simulink model "DCAC"  (R2020b)
settings: Solver=FixedStepDiscrete  StartTime=0.0  StopTime=0.05  FixedStep=1e-8  RelTol=1e-3
PreLoadFcn:
  | addpath("Sim\");
  | run(Sim_PreLoad_DCAC.mlx);
values from neighbouring files (symbols this model uses):
  C = 1/(wl*wl*L)    [BodeCalculation.m]
  L = sqrt(((w1*(Uo_*Uo_)/(wl*wl)) + (w1*w1*w1*(Uo_*Uo_)/(wl*wl*wl*wl))) / (w1*(Io_*Io_)))    [BodeCalculation.m]    (also in draw.m = sqrt(((w1 .* (Uo_ .^ 2) / (wl * wl)) + (w1 * w1 * w1 .* (Uo_)
undefined symbols (not defined in the file or in its folder): R_Load, Ts, V_DC
libraries: powerlib x22, powerlib_meascontrol x2, simulink x1
settings Model: Creator=VanillaC  LastModifiedBy=VanillaC
settings DataIOCC: ReturnWorkspaceOutputs=off
settings OptimizationCC: DefaultParameterBehavior=Inlined  EnhancedBackFolding=on  PassReuseOutputArgsAs=Individual arguments  ZeroExternalMemoryAtStartup=off  ZeroInternalMemoryAtStartup=off  OptimizeBlockOrder=speed  DifferentSizesBufferReuse=on  OptimizationCustomize=off  EfficientTunableParamExpr=on
settings DebuggingCC: ParameterTunabilityLossMsg=error  UnconnectedInputMsg=none  UnconnectedOutputMsg=none  UnconnectedLineMsg=none
settings ModelReferenceCC: EnableRefExpFcnMdlSchedulingChecks=off
settings SFSimCC: MATLABDynamicMemAlloc=off
settings RTWCC: Description=Embedded Coder  SystemTargetFile=ert.tlc  GenCodeOnly=on  TemplateMakefile=ert_default_tmf
settings CodeAppCC: ForceParamTrailComments=on  IgnoreCustomStorageClasses=off  OperatorAnnotations=on  SimulinkDataObjDesc=on  SFDataObjDesc=on  InsertBlockDesc=on  MATLABSourceComments=on
settings ERTTargetCC: TargetLangStandard=C99 (ISO)  GenerateSampleERTMain=on  SupportContinuousTime=on  InlinedParameterPlacement=NonHierarchical  ERTCustomFileTemplate=example_file_process.tlc

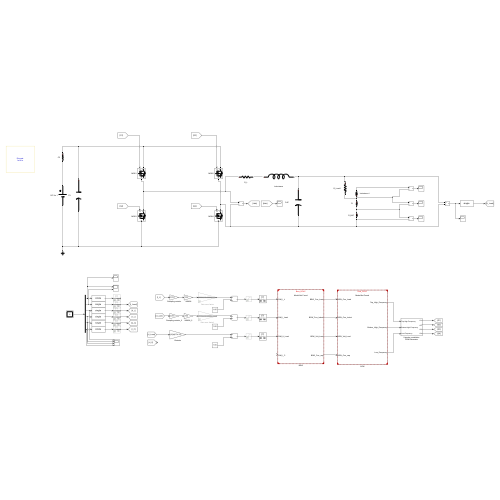
[thumbnail: Simulink's stored preview of the top-level diagram]
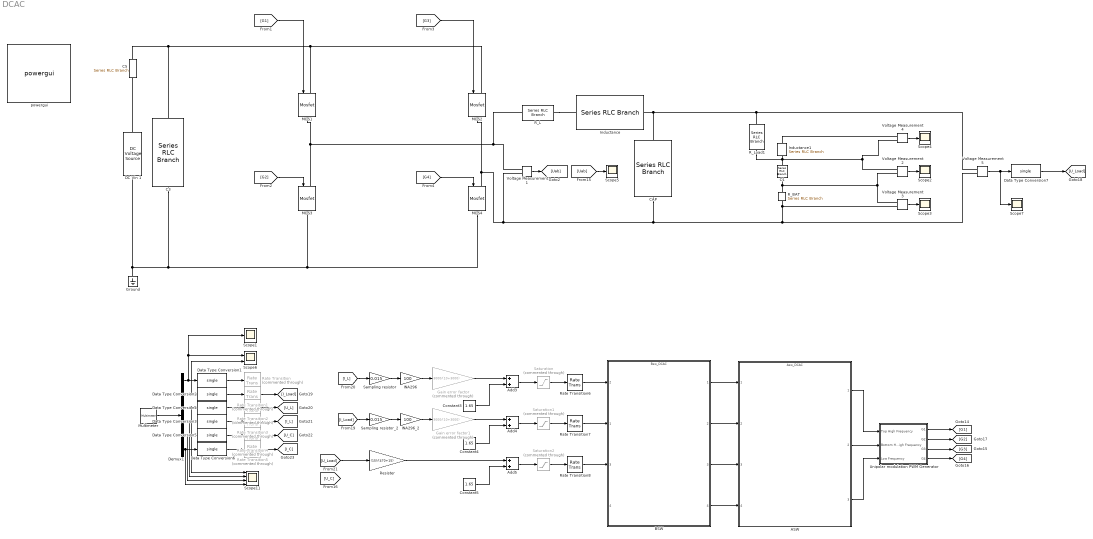
== system DCAC ==
  ASW : ModelReference  ModelNameDialog=Asw_DCAC.slx  SimulationMode=Normal  ModelReferenceVersion=1.140
  Add3 : Sum
  Add4 : Sum
  Add5 : Sum
  BSW : ModelReference  ModelNameDialog=Bsw_DCAC.slx  SimulationMode=Normal  ModelReferenceVersion=1.11
      settings: PortSchema="{\"entries\":[{\"content\":{\"sides\":[{\"content\":{\"connectorIds\":[\"In2\",\"In1\",\"In3\",\"In4\"]},\"type\":\"ConnectorPlacement.EquallySpacedRectSide\",\"uuid\":\"b2b7a57c-7cf1-4c06-9e54-7dc01d62324f\"},{\"content\":{\"connectorIds\":[\"Out1\",\"Out2\",\"Out3\",\"Out4\"],\"side\":\"RIGHT\"},\"type\":\"ConnectorPlacement.EquallySpacedRectSide\",\"uuid\":\"58967db2-deee-4275-8865-8f1f6f5d01b9\"},{\"content\":{\"side\":\"TOP\"},\"type\":\"ConnectorPlacement.EquallySpacedRectSide\",\"uuid\":\"d9088037-5ecd-44ee-9dae-30c0aa6e59e3\"}]},\"type\":\"ConnectorPlacement.EquallySpacedConnector\",\"uuid\":\"be37a7a2-a861-4ca5-b50a-1f8ecf43409b\"}],\"packageUris\":[\"http://schema.mathworks.com/mf0/Connector/R2020b\"],\"version\":\"1.0\"}"
  C1 : powerlib/Elements/Series RLC Branch  LConnTagsString=__new0  RConnTagsString=__new0  BranchType=C  Resistance=1000  Inductance=1e-3  SetiL0=off  InitialCurrent=0  Capacitance=2e-6  Setx0=off  InitialVoltage=0  Measurements=None
  C3 : powerlib/Elements/Series RLC Branch  LConnTagsString=__new0  RConnTagsString=__new0  BranchType=C  Resistance=1e-9  Inductance=1e-3  SetiL0=off  InitialCurrent=0  Capacitance=2.2e-3  Setx0=off  InitialVoltage=0  Measurements=None
  C5 : powerlib/Elements/Series RLC Branch  LConnTagsString=__new0  RConnTagsString=__new0  BranchType=R  Resistance=1e-9  Inductance=1e-3  SetiL0=off  InitialCurrent=0  Capacitance=2.2e-3  Setx0=off  InitialVoltage=0  Measurements=None
  CAP : powerlib/Elements/Series RLC Branch  LConnTagsString=__new0  RConnTagsString=__new0  BranchType=C  Resistance=1000  Inductance=1e-3  SetiL0=off  InitialCurrent=0  Capacitance=C  Setx0=off  InitialVoltage=0  Measurements=Branch voltage and current
  Constant3 : Constant  Value=1.65  OutDataTypeStr=single  SampleTime=-1
  Constant4 : Constant  Value=1.65  OutDataTypeStr=single  SampleTime=-1
  Constant5 : Constant  Value=1.65  OutDataTypeStr=single  SampleTime=-1
  DC Vin 1 : powerlib/Electrical Sources/DC Voltage Source  Amplitude=V_DC  Measurements=None
  Data Type Conversion{1..7} (7 alike) : DataTypeConversion  OutDataTypeStr=single
  Demux1 : Demux  Outputs=6
  Gain error factor : Gain  Commented=through  Gain=3000/(10+3000)
  Gain error factor1 : Gain  Commented=through  Gain=3000/(10+3000)
  Ground : powerlib/Elements/Ground  LConnTagsString=a
  INA296 : Gain  Gain=100
  INA296_2 : Gain  Gain=100
  Inductance : powerlib/Elements/Series RLC Branch  LConnTagsString=__new0  RConnTagsString=__new0  BranchType=L  Resistance=0.005  Inductance=L  SetiL0=off  InitialCurrent=0  Capacitance=470e-6  Setx0=off  InitialVoltage=0  Measurements=Branch voltage and current
  Inductance1 : powerlib/Elements/Series RLC Branch  LConnTagsString=__new0  RConnTagsString=__new0  BranchType=L  Resistance=0.005  Inductance=1.25e-3  SetiL0=off  InitialCurrent=0  Capacitance=470e-6  Setx0=off  InitialVoltage=0  Measurements=Branch voltage and current
  MOS1 : powerlib/Power Electronics/Mosfet  Ron=15e-3  Lon=0  Rd=0.01  Vfd=0.7  IC=0  Rs=1e5  Cs=inf  Measurements=off
  MOS2 : powerlib/Power Electronics/Mosfet  Ron=43e-3  Lon=0  Rd=0.01  Vfd=0.7  IC=0  Rs=1e5  Cs=inf  Measurements=off
  MOS3 : powerlib/Power Electronics/Mosfet  Ron=43e-3  Lon=0  Rd=0.01  Vfd=0.7  IC=0  Rs=1e5  Cs=inf  Measurements=off
  MOS4 : powerlib/Power Electronics/Mosfet  Ron=43e-3  Lon=0  Rd=0.01  Vfd=0.7  IC=0  Rs=1e5  Cs=inf  Measurements=off
  Multimeter : powerlib/Measurements/Multimeter  L=8  sel=[4 8 2 6 1 5]  yselected={}  Gain=[1 1 1 1 1 1]  OutputType=Complex  PlotAtSimulationStop=off  PhasorSimulation=off
  R_BAT : powerlib/Elements/Series RLC Branch  LConnTagsString=__new0  RConnTagsString=__new0  BranchType=R  Resistance=0.04  Inductance=1e-3  SetiL0=off  InitialCurrent=0  Capacitance=470e-6  Setx0=off  InitialVoltage=0  Measurements=None
  R_L : powerlib/Elements/Series RLC Branch  LConnTagsString=__new0  RConnTagsString=__new0  BranchType=R  Resistance=0.0005  Inductance=1e-3  SetiL0=off  InitialCurrent=0  Capacitance=470e-6  Setx0=off  InitialVoltage=0  Measurements=None
  R_Load1 : powerlib/Elements/Series RLC Branch  LConnTagsString=__new0  RConnTagsString=__new0  BranchType=R  Resistance=R_Load  Inductance=1e-3  SetiL0=off  InitialCurrent=0  Capacitance=470e-6  Setx0=off  InitialVoltage=0  Measurements=Branch voltage and current
  Rate Transition{,1..5} (6 alike) : RateTransition  Commented=through  OutPortSampleTime=Ts
  Rate Transition6 : RateTransition  OutPortSampleTime=Ts
  Rate Transition7 : RateTransition  OutPortSampleTime=Ts
  Rate Transition8 : RateTransition  OutPortSampleTime=Ts
  Resister : Gain  Gain=(15)/(470+15)
  Sampling resistor : Gain  Gain=0.015
  Sampling resistor_2 : Gain  Gain=0.015
  Saturation : Saturate  Commented=through  UpperLimit=3.3  LowerLimit=0
  Saturation1 : Saturate  Commented=through  UpperLimit=3.3  LowerLimit=0
  Saturation2 : Saturate  Commented=through  UpperLimit=3.3  LowerLimit=0
  Scope{1..5,7} (6 alike) : Scope
  Scope11 : Scope  NumInputPorts=4
  Scope6 : Scope  NumInputPorts=2
  Unipolar modulation PWM Generator : Subsystem
  Voltage Measurement{1..5} (5 alike) : powerlib/Measurements/Voltage Measurement  PhasorSimulation=off  OutputType=Complex  PSBequivalent=0
  powergui : powerlib/powergui  Priority=1  SimulationMode=Discrete  SampleTime=1e-8  frequency=60  Iterations=50  frequencyindice=0  Pbase=100e6  ErrMax=1e-4  UnitsV=kV  UnitsW=MW  buscounter=0  FunctionMessages=off  echomessages=off  EnableUseOfTLC=off  CurrentSourceSwitches=off  DisableSnubberDevices=off  DisableRonSwitches=off  DisableVfSwitches=off  DisplayEquations=off  AutomaticDiscreteSolvers=off  SolverType=Tustin/Backward Euler (TBE)  Interpol=off  ExternalGateDelay=off  methode=off  Ts=100  x0status=blocks  SPID=on  SwTol=0  HookPort=off  NonlinearTolerance=1e-4  nMaxIteration=100  ContinueOnMaxIteration=off  RestoreLinks=warning  ResistiveCurrentMeasurement=off  Frange=[0:2:500]  Ylog=off  Xlog=on  ShowGrid=off  save=off  variable=ZData  structure=0  ZoomFFT=off  StartTime=0.0  cycles=1  DisplayStyle=1  fundamental=60  FreqAxis=off  MaxFrequency=1000  frequencyindicesteady=1  RmsSteady=1  display=off
  wires:
  [G3] -> MOS2/1
  [G4] -> MOS4/1
  [G2] -> MOS3/1
  [G1] -> MOS1/1
  Voltage Measurement1/1 -> [Uab]
  Unipolar modulation PWM Generator/2(G2) -> [G2]
  Unipolar modulation PWM Generator/1(G1) -> [G1]
  Unipolar modulation PWM Generator/4(G4) -> [G4]
  Unipolar modulation PWM Generator/3(G3) -> [G3]
  ASW/1 -> Unipolar modulation PWM Generator/1(Top High Frequency)
  ASW/2 -> Unipolar modulation PWM Generator/2(Bottom High Frequency)
  ASW/3 -> Unipolar modulation PWM Generator/3(Low Frequency)
  Multimeter/1 -> Demux1/1
  Demux1/1 -> Scope6/1, Scope1/1, Data Type Conversion1/1
  Demux1/2 -> Scope6/2, Data Type Conversion2/1
  Demux1/3 -> Scope11/1, Data Type Conversion4/1
  Demux1/4 -> Scope11/2, Data Type Conversion3/1
  Data Type Conversion1/1 -> Rate Transition/1
  Data Type Conversion2/1 -> Rate Transition1/1
  Data Type Conversion3/1 -> Rate Transition3/1
  Data Type Conversion4/1 -> Rate Transition2/1
  Rate Transition1/1 -> [I_Load]
  Rate Transition2/1 -> [U_L]
  Rate Transition3/1 -> [I_L]
  Rate Transition4/1 -> [U_C]
  Data Type Conversion5/1 -> Rate Transition4/1
  Data Type Conversion6/1 -> Rate Transition5/1
  Rate Transition5/1 -> [I_C]
  Demux1/5 -> Scope11/3, Data Type Conversion5/1
  [I_L] -> Sampling resistor/1
  Demux1/6 -> Scope11/4, Data Type Conversion6/1
  [I_Load] -> Sampling resistor_2/1
  Sampling resistor/1 -> INA296/1
  Sampling resistor_2/1 -> INA296_2/1
  Add3/1 -> Saturation/1
  Constant3/1 -> Add3/2
  Gain error factor/1 -> Add3/1
  INA296/1 -> Gain error factor/1
  Add4/1 -> Saturation1/1
  Constant4/1 -> Add4/2
  Gain error factor1/1 -> Add4/1
  INA296_2/1 -> Gain error factor1/1
  Saturation/1 -> Rate Transition6/1
  Saturation1/1 -> Rate Transition7/1
  Constant5/1 -> Add5/2
  Resister/1 -> Add5/1
  Add5/1 -> Saturation2/1
  Rate Transition6/1 -> BSW/2
  Rate Transition7/1 -> BSW/1
  Rate Transition8/1 -> BSW/3
  BSW/1 -> ASW/1
  BSW/2 -> ASW/2
  BSW/3 -> ASW/3
  BSW/4 -> ASW/4
  Saturation2/1 -> Rate Transition8/1
  [Uab] -> Scope5/1
  [U_Load] -> Resister/1
  Voltage Measurement2/1 -> Scope2/1
  Voltage Measurement3/1 -> Scope3/1
  Voltage Measurement4/1 -> Scope4/1
  Voltage Measurement5/1 -> Scope7/1, Data Type Conversion7/1
  Data Type Conversion7/1 -> [U_Load]
  connections:
  R_L/LConn1 -- Voltage Measurement1/LConn1 -- MOS1/RConn1 -- MOS3/LConn1
  C3/LConn1 -- C5/LConn1 -- MOS1/LConn1 -- MOS2/LConn1
  DC Vin 1/RConn1 -- C5/RConn1
  C3/RConn1 -- Ground/LConn1 -- DC Vin 1/LConn1 -- MOS4/RConn1 -- MOS3/RConn1
  R_BAT/LConn1 -- C1/RConn1 -- Voltage Measurement2/LConn2 -- Voltage Measurement3/LConn1
  R_L/RConn1 -- Inductance/LConn1
  CAP/LConn1 -- Voltage Measurement5/LConn1 -- R_Load1/LConn1 -- Inductance/RConn1
  MOS2/RConn1 -- Voltage Measurement1/LConn2 -- Voltage Measurement5/LConn2 -- R_BAT/RConn1 -- Voltage Measurement3/LConn2 -- CAP/RConn1 -- MOS4/LConn1
  Voltage Measurement2/LConn1 -- R_Load1/RConn1 -- C1/LConn1 -- Inductance1/LConn1 -- Voltage Measurement4/LConn2
  Voltage Measurement4/LConn1 -- Inductance1/RConn1

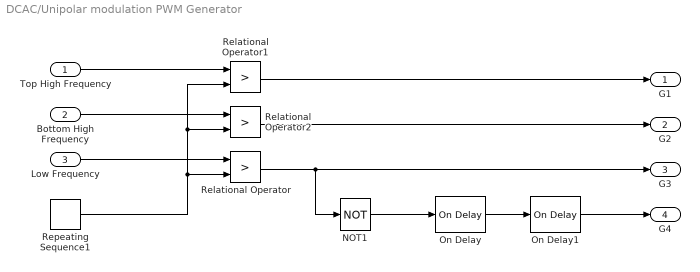
== system DCAC/Unipolar modulation PWM Generator ==
  Top High Frequency : Inport
  Bottom High Frequency : Inport  Port=2
  Low Frequency : Inport  Port=3
  NOT1 : Logic  Operator=NOT  IconShape=distinctive  AllPortsSameDT=off  OutDataTypeStr=boolean
  On Delay : powerlib_meascontrol/Logic/On Delay  DelayType=On delay  delay=10e-9  ic=0  Ts=0
  On Delay1 : powerlib_meascontrol/Logic/On Delay  DelayType=Off delay  delay=10e-9  ic=0  Ts=0
  Relational Operator : RelationalOperator  Operator=>  OutDataTypeStr=boolean  RndMeth=Simplest
  Relational Operator1 : RelationalOperator  Operator=>  OutDataTypeStr=boolean  RndMeth=Simplest
  Relational Operator2 : RelationalOperator  Operator=>  OutDataTypeStr=boolean  RndMeth=Simplest
  Repeating Sequence1 : simulink/Sources/Repeating Sequence  rep_seq_t=[0 Ts/2 Ts]  rep_seq_y=[0 1 0]
  G1 : Outport
  G2 : Outport  Port=2
  G3 : Outport  Port=3
  G4 : Outport  Port=4
  wires:
  Repeating Sequence1/1 -> Relational Operator/2, Relational Operator2/2, Relational Operator1/2
  NOT1/1 -> On Delay/1
  Relational Operator/1 -> G3/1, NOT1/1
  Relational Operator1/1 -> G1/1
  Top High Frequency/1 -> Relational Operator1/1
  Relational Operator2/1 -> G2/1
  Bottom High Frequency/1 -> Relational Operator2/1
  Low Frequency/1 -> Relational Operator/1
  On Delay/1 -> On Delay1/1
  On Delay1/1 -> G4/1
